simulink model "Exp3"  (R2020a)
settings: Solver=VariableStepAuto  StartTime=0.0  StopTime=100  RelTol=1e-3
InitFcn:
  | Voc=32.9;
  | Iscn=8.21;
  | k=1.38e-23;
  | Ns=54;
  | Np=1;
  | G1=1000;
  | G2=800;
  | G3=600;
  | Gn=1000;
  | Kv=-0.1230;
  | KI=0.0032;
  | T=301;
  | Tn=300;
  | q=1.6e-19;
  | n=1;
  | I0n=9.85e-8;
  | Eg=1.12;
  | Ign=8.214;
  | Rs=0.221;
  | Rp=414.5;
  | a=1.0
libraries: powerlib x19, simulink x1
settings Model: Creator=ahmed  LastModifiedBy=ahmed
settings DataIOCC: Refine=250

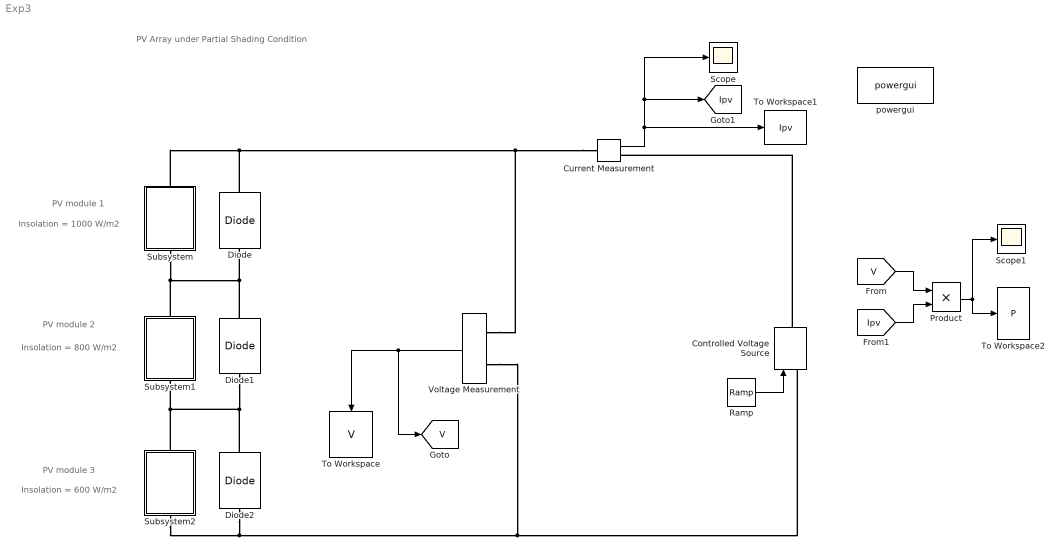
== system Exp3 ==
  note: PV Array under Partial Shading Condition
  note: Insolation = 1000 W/m2
  note: PV module 1
  note: PV module 2
  note: PV module 3
  note: Insolation = 800 W/m2
  note: Insolation = 600 W/m2
  Controlled Voltage Source : powerlib/Electrical Sources/Controlled Voltage Source  Initialize=on  Source_Type=AC  Amplitude=0  Phase=0  Frequency=0  Measurements=None
  Current Measurement : powerlib/Measurements/Current Measurement  PhasorSimulation=off  OutputType=Complex  PSBequivalent=0
  Diode : powerlib/Power Electronics/Diode  Ron=0.001  Lon=0  Vf=0.8  IC=0  UseSnubber=0  Rs=500  Cs=250e-9  Measurements=off
  Diode1 : powerlib/Power Electronics/Diode  Ron=0.001  Lon=0  Vf=0.8  IC=0  UseSnubber=0  Rs=500  Cs=250e-9  Measurements=off
  Diode2 : powerlib/Power Electronics/Diode  Ron=0.001  Lon=0  Vf=0.8  IC=0  UseSnubber=0  Rs=500  Cs=250e-9  Measurements=off
  Product : Product
  Ramp : simulink/Sources/Ramp  slope=1  start=0  InitialOutput=0
  Scope : Scope
  Scope1 : Scope
  Subsystem : Subsystem
  Subsystem1 : Subsystem
  Subsystem2 : Subsystem
  To Workspace : ToWorkspace  VariableName=V  SaveFormat=Timeseries  SampleTime=-1
  To Workspace1 : ToWorkspace  VariableName=Ipv  SaveFormat=Timeseries  SampleTime=-1
  To Workspace2 : ToWorkspace  VariableName=P  SaveFormat=Timeseries  SampleTime=-1
  Voltage Measurement : powerlib/Measurements/Voltage Measurement  PhasorSimulation=off  OutputType=Complex  PSBequivalent=0
  powergui : powerlib/powergui  Priority=1  SimulationMode=Continuous  SampleTime=50e-6  frequency=60  Iterations=50  frequencyindice=0  Pbase=100e6  ErrMax=1e-4  UnitsV=kV  UnitsW=MW  buscounter=0  FunctionMessages=off  echomessages=off  EnableUseOfTLC=off  CurrentSourceSwitches=off  DisableSnubberDevices=off  DisableRonSwitches=off  DisableVfSwitches=off  DisplayEquations=off  AutomaticDiscreteSolvers=off  SolverType=Tustin/Backward Euler (TBE)  Interpol=off  ExternalGateDelay=off  methode=off  Ts=100  x0status=blocks  SPID=on  SwTol=0  HookPort=off  NonlinearTolerance=1e-4  nMaxIteration=100  ContinueOnMaxIteration=off  RestoreLinks=warning  ResistiveCurrentMeasurement=off  Frange=[0:2:500]  Ylog=off  Xlog=on  ShowGrid=off  save=off  variable=ZData  structure=0  ZoomFFT=off  StartTime=0.0  cycles=1  DisplayStyle=1  fundamental=60  FreqAxis=off  MaxFrequency=1000  frequencyindicesteady=1  RmsSteady=1  display=off
  tag scope: Ipv=global, V=global
  wires:
  Ramp/1 -> Controlled Voltage Source/1
  Voltage Measurement/1 -> [V], To Workspace/1
  Current Measurement/1 -> To Workspace1/1, [Ipv], Scope/1
  [V] -> Product/1
  [Ipv] -> Product/2
  Product/1 -> Scope1/1, To Workspace2/1
  connections:
  Current Measurement/LConn1 -- Diode/RConn1 -- Subsystem/RConn1 -- Voltage Measurement/LConn1
  Controlled Voltage Source/RConn1 -- Current Measurement/RConn1
  Controlled Voltage Source/LConn1 -- Diode2/LConn1 -- Subsystem2/LConn1 -- Voltage Measurement/LConn2
  Subsystem2/RConn1 -- Diode2/RConn1 -- Diode1/LConn1 -- Subsystem1/LConn1
  Subsystem/LConn1 -- Subsystem1/RConn1 -- Diode/LConn1 -- Diode1/RConn1

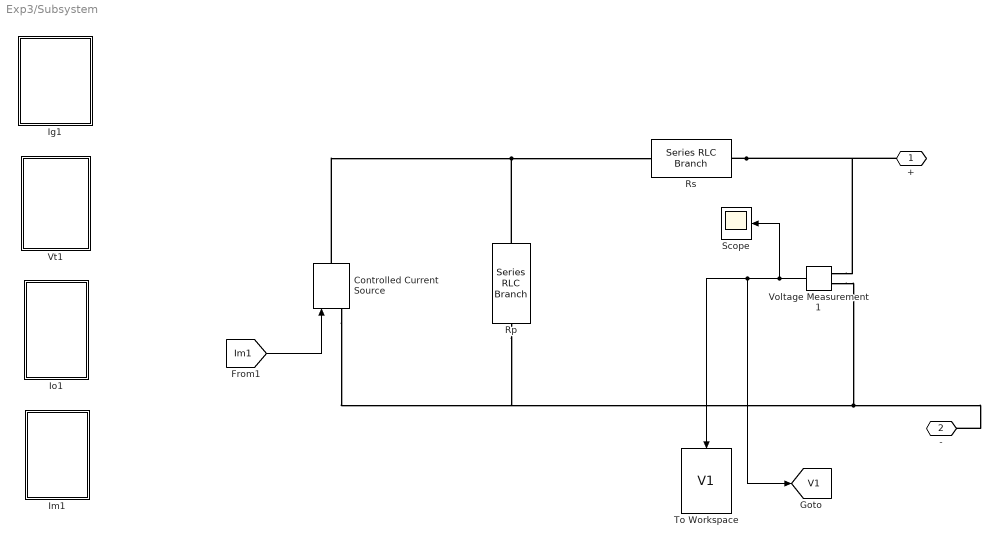
== system Exp3/Subsystem ==
  Controlled Current Source : powerlib/Electrical Sources/Controlled Current Source  Initialize=on  Source_Type=AC  Amplitude=0  Phase=0  Frequency=0  Measurements=None
  Ig1 : Subsystem
  Im1 : Subsystem
  Io1 : Subsystem
  Rp : powerlib/Elements/Series RLC Branch  LConnTagsString=__new0  RConnTagsString=__new0  BranchType=R  Resistance=Rp  Inductance=1e-3  SetiL0=off  InitialCurrent=0  Capacitance=1e-6  Setx0=off  InitialVoltage=0  Measurements=None
  Rs : powerlib/Elements/Series RLC Branch  LConnTagsString=__new0  RConnTagsString=__new0  BranchType=R  Resistance=Rs  Inductance=1e-3  SetiL0=off  InitialCurrent=0  Capacitance=1e-6  Setx0=off  InitialVoltage=0  Measurements=None
  Scope : Scope
  To Workspace : ToWorkspace  VariableName=V1  SaveFormat=Timeseries  SampleTime=-1
  Voltage Measurement1 : powerlib/Measurements/Voltage Measurement  PhasorSimulation=off  OutputType=Complex  PSBequivalent=0
  Vt1 : Subsystem
  + : PMIOPort  Side=Right
  - : PMIOPort  Port=2  Side=Left
  tag scope: V1=global
  wires:
  [Im1] -> Controlled Current Source/1
  Voltage Measurement1/1 -> [V1], To Workspace/1, Scope/1
  connections:
  Rs/RConn1 -- +/RConn1 -- Voltage Measurement1/LConn1
  Voltage Measurement1/LConn2 -- Controlled Current Source/LConn1 -- Rp/RConn1 -- -/RConn1
  Rp/LConn1 -- Controlled Current Source/RConn1 -- Rs/LConn1

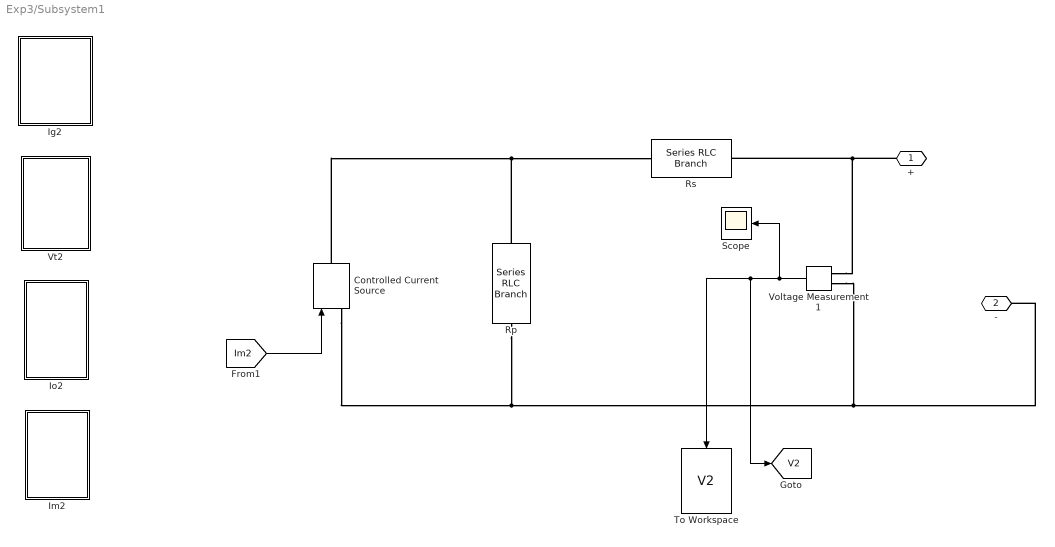
== system Exp3/Subsystem1 ==
  Controlled Current Source : powerlib/Electrical Sources/Controlled Current Source  Initialize=on  Source_Type=AC  Amplitude=0  Phase=0  Frequency=0  Measurements=None
  Ig2 : Subsystem
  Im2 : Subsystem
  Io2 : Subsystem
  Rp : powerlib/Elements/Series RLC Branch  LConnTagsString=__new0  RConnTagsString=__new0  BranchType=R  Resistance=Rp  Inductance=1e-3  SetiL0=off  InitialCurrent=0  Capacitance=1e-6  Setx0=off  InitialVoltage=0  Measurements=None
  Rs : powerlib/Elements/Series RLC Branch  LConnTagsString=__new0  RConnTagsString=__new0  BranchType=R  Resistance=Rs  Inductance=1e-3  SetiL0=off  InitialCurrent=0  Capacitance=1e-6  Setx0=off  InitialVoltage=0  Measurements=None
  Scope : Scope
  To Workspace : ToWorkspace  VariableName=V2  SaveFormat=Timeseries  SampleTime=-1
  Voltage Measurement1 : powerlib/Measurements/Voltage Measurement  PhasorSimulation=off  OutputType=Complex  PSBequivalent=0
  Vt2 : Subsystem
  + : PMIOPort  Side=Right
  - : PMIOPort  Port=2  Side=Left
  tag scope: V2=global
  wires:
  Voltage Measurement1/1 -> Scope/1, [V2], To Workspace/1
  [Im2] -> Controlled Current Source/1
  connections:
  Controlled Current Source/RConn1 -- Rp/LConn1 -- Rs/LConn1
  -/RConn1 -- Voltage Measurement1/LConn2 -- Rp/RConn1 -- Controlled Current Source/LConn1
  +/RConn1 -- Rs/RConn1 -- Voltage Measurement1/LConn1

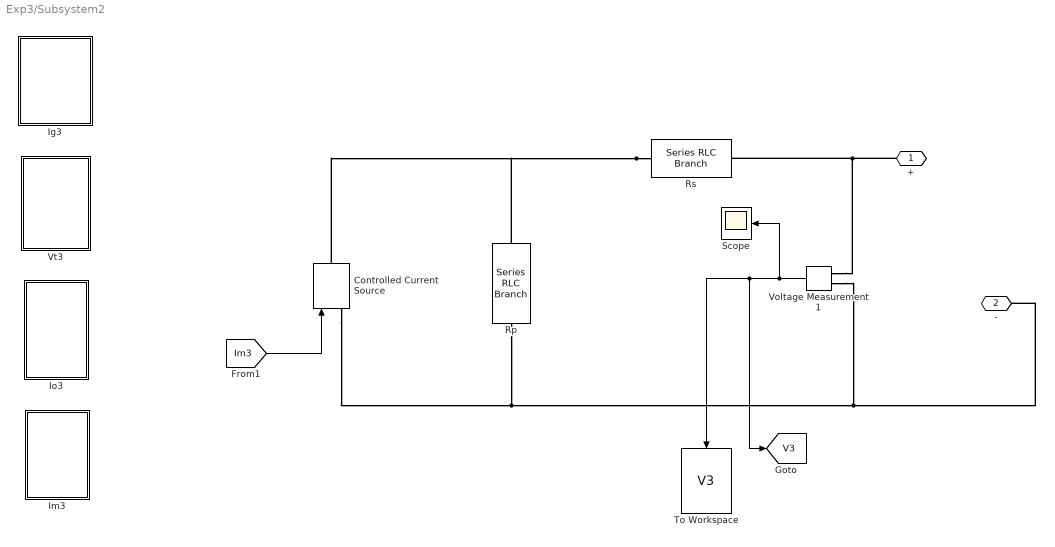
== system Exp3/Subsystem2 ==
  Controlled Current Source : powerlib/Electrical Sources/Controlled Current Source  Initialize=on  Source_Type=AC  Amplitude=0  Phase=0  Frequency=0  Measurements=None
  Ig3 : Subsystem
  Im3 : Subsystem
  Io3 : Subsystem
  Rp : powerlib/Elements/Series RLC Branch  LConnTagsString=__new0  RConnTagsString=__new0  BranchType=R  Resistance=Rp  Inductance=1e-3  SetiL0=off  InitialCurrent=0  Capacitance=1e-6  Setx0=off  InitialVoltage=0  Measurements=None
  Rs : powerlib/Elements/Series RLC Branch  LConnTagsString=__new0  RConnTagsString=__new0  BranchType=R  Resistance=Rs  Inductance=1e-3  SetiL0=off  InitialCurrent=0  Capacitance=1e-6  Setx0=off  InitialVoltage=0  Measurements=None
  Scope : Scope
  To Workspace : ToWorkspace  VariableName=V3  SaveFormat=Timeseries  SampleTime=-1
  Voltage Measurement1 : powerlib/Measurements/Voltage Measurement  PhasorSimulation=off  OutputType=Complex  PSBequivalent=0
  Vt3 : Subsystem
  + : PMIOPort  Side=Right
  - : PMIOPort  Port=2  Side=Left
  tag scope: V3=global
  wires:
  [Im3] -> Controlled Current Source/1
  Voltage Measurement1/1 -> To Workspace/1, [V3], Scope/1
  connections:
  Voltage Measurement1/LConn1 -- Rs/RConn1 -- +/RConn1
  Controlled Current Source/LConn1 -- Rp/RConn1 -- Voltage Measurement1/LConn2 -- -/RConn1
  Rs/LConn1 -- Rp/LConn1 -- Controlled Current Source/RConn1

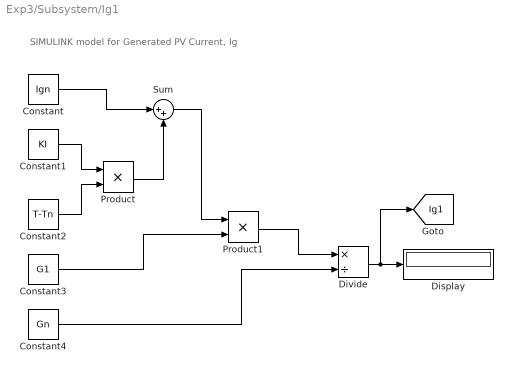
== system Exp3/Subsystem/Ig1 ==
  note: SIMULINK model for Generated PV Current, Ig
  Constant : Constant  Value=Ign
  Constant1 : Constant  Value=KI
  Constant2 : Constant  Value=T-Tn
  Constant3 : Constant  Value=G1
  Constant4 : Constant  Value=Gn
  Display : Display
  Divide : Product  Inputs=*/
  Product : Product
  Product1 : Product
  Sum : Sum  Inputs=|++
  tag scope: Ig1=global
  wires:
  Divide/1 -> [Ig1], Display/1
  Product1/1 -> Divide/1
  Constant1/1 -> Product/1
  Constant/1 -> Sum/1
  Product/1 -> Sum/2
  Constant2/1 -> Product/2
  Constant3/1 -> Product1/2
  Sum/1 -> Product1/1
  Constant4/1 -> Divide/2

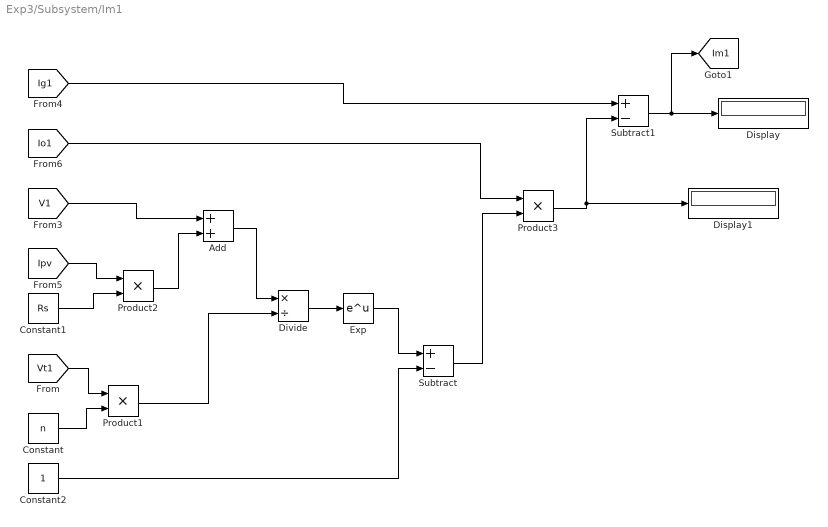
== system Exp3/Subsystem/Im1 ==
  Add : Sum
  Constant : Constant  Value=n
  Constant1 : Constant  Value=Rs
  Constant2 : Constant
  Display : Display
  Display1 : Display
  Divide : Product  Inputs=*/
  Exp : Math  SaturateOnIntegerOverflow=on
  Product1 : Product
  Product2 : Product
  Product3 : Product
  Subtract : Sum  Inputs=+-
  Subtract1 : Sum  Inputs=+-
  tag scope: Im1=global
  wires:
  Exp/1 -> Subtract/1
  Product2/1 -> Add/2
  [Vt1] -> Product1/1
  [Ig1] -> Subtract1/1
  Constant1/1 -> Product2/2
  Subtract1/1 -> [Im1], Display/1
  Add/1 -> Divide/1
  [Ipv] -> Product2/1
  Product1/1 -> Divide/2
  [V1] -> Add/1
  [Io1] -> Product3/1
  Divide/1 -> Exp/1
  Constant2/1 -> Subtract/2
  Subtract/1 -> Product3/2
  Product3/1 -> Display1/1, Subtract1/2
  Constant/1 -> Product1/2

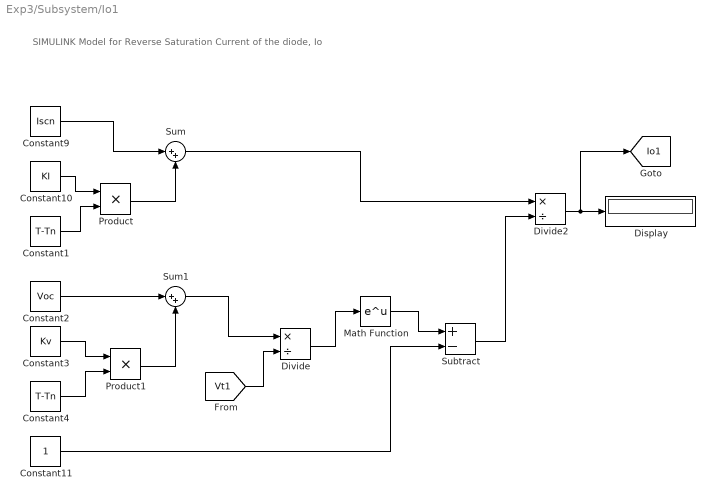
== system Exp3/Subsystem/Io1 ==
  note: SIMULINK Model for Reverse Saturation Current of the diode, Io
  Constant1 : Constant  Value=T-Tn
  Constant10 : Constant  Value=KI
  Constant11 : Constant
  Constant2 : Constant  Value=Voc
  Constant3 : Constant  Value=Kv
  Constant4 : Constant  Value=T-Tn
  Constant9 : Constant  Value=Iscn
  Display : Display
  Divide : Product  Inputs=*/
  Divide2 : Product  Inputs=*/
  Math Function : Math  SaturateOnIntegerOverflow=on
  Product : Product
  Product1 : Product
  Subtract : Sum  Inputs=+-
  Sum : Sum  Inputs=|++
  Sum1 : Sum  Inputs=|++
  tag scope: Io1=global
  wires:
  Constant4/1 -> Product1/2
  [Vt1] -> Divide/2
  Product/1 -> Sum/2
  Math Function/1 -> Subtract/1
  Sum/1 -> Divide2/1
  Constant9/1 -> Sum/1
  Product1/1 -> Sum1/2
  Constant11/1 -> Subtract/2
  Constant3/1 -> Product1/1
  Sum1/1 -> Divide/1
  Divide2/1 -> [Io1], Display/1
  Constant10/1 -> Product/1
  Subtract/1 -> Divide2/2
  Constant2/1 -> Sum1/1
  Divide/1 -> Math Function/1
  Constant1/1 -> Product/2

== system Exp3/Subsystem/Vt1 ==
  note: SIMULINK model for Temparature Equivalent Voltage, Vt
  Constant5 : Constant  Value=Ns
  Constant6 : Constant  Value=k
  Constant7 : Constant  Value=T
  Constant8 : Constant  Value=q
  Display1 : Display
  Divide1 : Product  Inputs=*/
  Product2 : Product  Inputs=3
  tag scope: Vt1=global
  wires:
  Product2/1 -> Divide1/1
  Divide1/1 -> [Vt1], Display1/1
  Constant5/1 -> Product2/1
  Constant7/1 -> Product2/3
  Constant8/1 -> Divide1/2
  Constant6/1 -> Product2/2

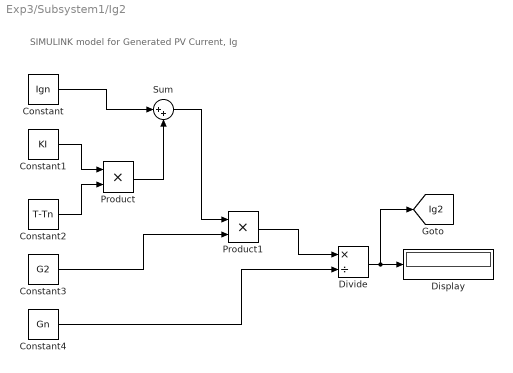
== system Exp3/Subsystem1/Ig2 ==
  note: SIMULINK model for Generated PV Current, Ig
  Constant : Constant  Value=Ign
  Constant1 : Constant  Value=KI
  Constant2 : Constant  Value=T-Tn
  Constant3 : Constant  Value=G2
  Constant4 : Constant  Value=Gn
  Display : Display
  Divide : Product  Inputs=*/
  Product : Product
  Product1 : Product
  Sum : Sum  Inputs=|++
  tag scope: Ig2=global
  wires:
  Constant4/1 -> Divide/2
  Sum/1 -> Product1/1
  Constant3/1 -> Product1/2
  Constant2/1 -> Product/2
  Product/1 -> Sum/2
  Constant/1 -> Sum/1
  Constant1/1 -> Product/1
  Product1/1 -> Divide/1
  Divide/1 -> Display/1, [Ig2]

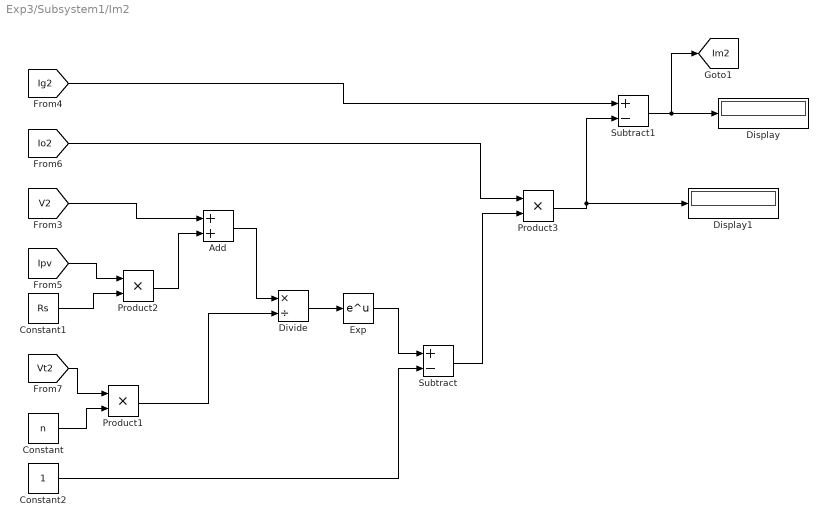
== system Exp3/Subsystem1/Im2 ==
  Add : Sum
  Constant : Constant  Value=n
  Constant1 : Constant  Value=Rs
  Constant2 : Constant
  Display : Display
  Display1 : Display
  Divide : Product  Inputs=*/
  Exp : Math  SaturateOnIntegerOverflow=on
  Product1 : Product
  Product2 : Product
  Product3 : Product
  Subtract : Sum  Inputs=+-
  Subtract1 : Sum  Inputs=+-
  tag scope: Im2=global
  wires:
  Constant/1 -> Product1/2
  Product3/1 -> Subtract1/2, Display1/1
  Subtract/1 -> Product3/2
  Constant2/1 -> Subtract/2
  Divide/1 -> Exp/1
  [Io2] -> Product3/1
  [V2] -> Add/1
  Product1/1 -> Divide/2
  [Ipv] -> Product2/1
  Add/1 -> Divide/1
  Subtract1/1 -> Display/1, [Im2]
  Constant1/1 -> Product2/2
  [Ig2] -> Subtract1/1
  [Vt2] -> Product1/1
  Product2/1 -> Add/2
  Exp/1 -> Subtract/1

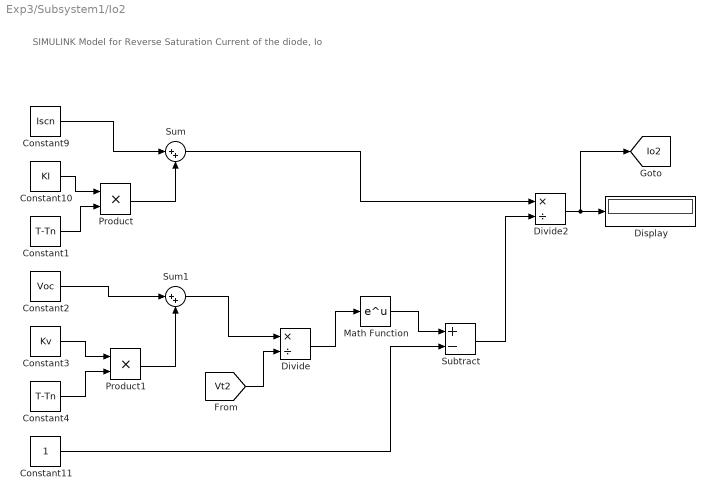
== system Exp3/Subsystem1/Io2 ==
  note: SIMULINK Model for Reverse Saturation Current of the diode, Io
  Constant1 : Constant  Value=T-Tn
  Constant10 : Constant  Value=KI
  Constant11 : Constant
  Constant2 : Constant  Value=Voc
  Constant3 : Constant  Value=Kv
  Constant4 : Constant  Value=T-Tn
  Constant9 : Constant  Value=Iscn
  Display : Display
  Divide : Product  Inputs=*/
  Divide2 : Product  Inputs=*/
  Math Function : Math  SaturateOnIntegerOverflow=on
  Product : Product
  Product1 : Product
  Subtract : Sum  Inputs=+-
  Sum : Sum  Inputs=|++
  Sum1 : Sum  Inputs=|++
  tag scope: Io2=global
  wires:
  Constant1/1 -> Product/2
  Divide/1 -> Math Function/1
  Constant2/1 -> Sum1/1
  Subtract/1 -> Divide2/2
  Constant10/1 -> Product/1
  Divide2/1 -> Display/1, [Io2]
  Sum1/1 -> Divide/1
  Constant3/1 -> Product1/1
  Constant11/1 -> Subtract/2
  Product1/1 -> Sum1/2
  Constant9/1 -> Sum/1
  Sum/1 -> Divide2/1
  Math Function/1 -> Subtract/1
  Product/1 -> Sum/2
  [Vt2] -> Divide/2
  Constant4/1 -> Product1/2

== system Exp3/Subsystem1/Vt2 ==
  note: SIMULINK model for Temparature Equivalent Voltage, Vt
  Constant5 : Constant  Value=Ns
  Constant6 : Constant  Value=k
  Constant7 : Constant  Value=T
  Constant8 : Constant  Value=q
  Display1 : Display
  Divide1 : Product  Inputs=*/
  Product2 : Product  Inputs=3
  tag scope: Vt2=global
  wires:
  Constant6/1 -> Product2/2
  Constant8/1 -> Divide1/2
  Constant7/1 -> Product2/3
  Constant5/1 -> Product2/1
  Divide1/1 -> Display1/1, [Vt2]
  Product2/1 -> Divide1/1

== system Exp3/Subsystem2/Ig3 ==
  note: SIMULINK model for Generated PV Current, Ig
  Constant : Constant  Value=Ign
  Constant1 : Constant  Value=KI
  Constant2 : Constant  Value=T-Tn
  Constant3 : Constant  Value=G3
  Constant4 : Constant  Value=Gn
  Display : Display
  Divide : Product  Inputs=*/
  Product : Product
  Product1 : Product
  Sum : Sum  Inputs=|++
  tag scope: Ig3=global
  wires:
  Divide/1 -> [Ig3], Display/1
  Product1/1 -> Divide/1
  Constant1/1 -> Product/1
  Constant/1 -> Sum/1
  Product/1 -> Sum/2
  Constant2/1 -> Product/2
  Constant3/1 -> Product1/2
  Sum/1 -> Product1/1
  Constant4/1 -> Divide/2

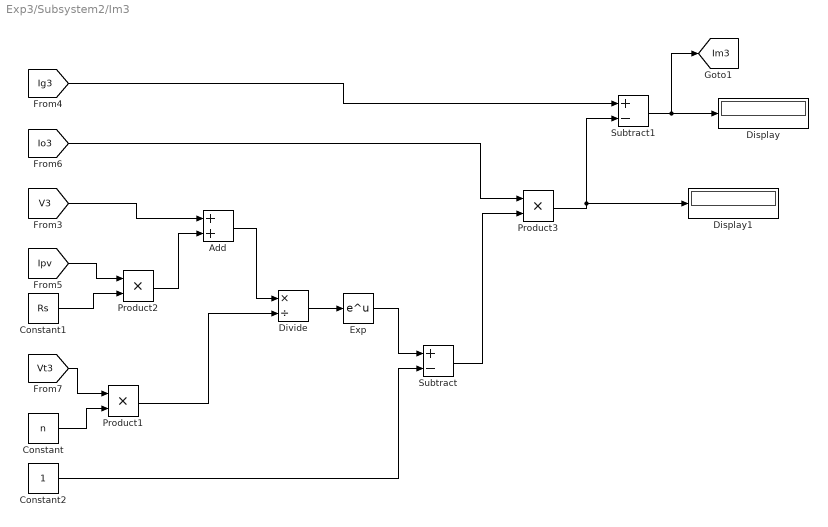
== system Exp3/Subsystem2/Im3 ==
  Add : Sum
  Constant : Constant  Value=n
  Constant1 : Constant  Value=Rs
  Constant2 : Constant
  Display : Display
  Display1 : Display
  Divide : Product  Inputs=*/
  Exp : Math  SaturateOnIntegerOverflow=on
  Product1 : Product
  Product2 : Product
  Product3 : Product
  Subtract : Sum  Inputs=+-
  Subtract1 : Sum  Inputs=+-
  tag scope: Im3=global
  wires:
  Exp/1 -> Subtract/1
  Product2/1 -> Add/2
  [Vt3] -> Product1/1
  [Ig3] -> Subtract1/1
  Constant1/1 -> Product2/2
  Subtract1/1 -> [Im3], Display/1
  Add/1 -> Divide/1
  [Ipv] -> Product2/1
  Product1/1 -> Divide/2
  [V3] -> Add/1
  [Io3] -> Product3/1
  Divide/1 -> Exp/1
  Constant2/1 -> Subtract/2
  Subtract/1 -> Product3/2
  Product3/1 -> Display1/1, Subtract1/2
  Constant/1 -> Product1/2

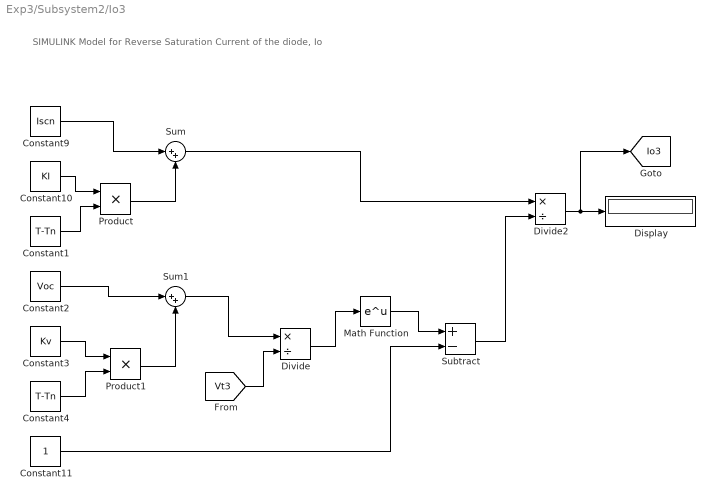
== system Exp3/Subsystem2/Io3 ==
  note: SIMULINK Model for Reverse Saturation Current of the diode, Io
  Constant1 : Constant  Value=T-Tn
  Constant10 : Constant  Value=KI
  Constant11 : Constant
  Constant2 : Constant  Value=Voc
  Constant3 : Constant  Value=Kv
  Constant4 : Constant  Value=T-Tn
  Constant9 : Constant  Value=Iscn
  Display : Display
  Divide : Product  Inputs=*/
  Divide2 : Product  Inputs=*/
  Math Function : Math  SaturateOnIntegerOverflow=on
  Product : Product
  Product1 : Product
  Subtract : Sum  Inputs=+-
  Sum : Sum  Inputs=|++
  Sum1 : Sum  Inputs=|++
  tag scope: Io3=global
  wires:
  Constant4/1 -> Product1/2
  [Vt3] -> Divide/2
  Product/1 -> Sum/2
  Math Function/1 -> Subtract/1
  Sum/1 -> Divide2/1
  Constant9/1 -> Sum/1
  Product1/1 -> Sum1/2
  Constant11/1 -> Subtract/2
  Constant3/1 -> Product1/1
  Sum1/1 -> Divide/1
  Divide2/1 -> [Io3], Display/1
  Constant10/1 -> Product/1
  Subtract/1 -> Divide2/2
  Constant2/1 -> Sum1/1
  Divide/1 -> Math Function/1
  Constant1/1 -> Product/2

== system Exp3/Subsystem2/Vt3 ==
  note: SIMULINK model for Temparature Equivalent Voltage, Vt
  Constant5 : Constant  Value=Ns
  Constant6 : Constant  Value=k
  Constant7 : Constant  Value=T
  Constant8 : Constant  Value=q
  Display1 : Display
  Divide1 : Product  Inputs=*/
  Product2 : Product  Inputs=3
  tag scope: Vt3=global
  wires:
  Product2/1 -> Divide1/1
  Divide1/1 -> [Vt3], Display1/1
  Constant5/1 -> Product2/1
  Constant7/1 -> Product2/3
  Constant8/1 -> Divide1/2
  Constant6/1 -> Product2/2
